simulink model "robot"  (R2014b)
settings: Solver=ode3  StartTime=0.0  StopTime=inf  RelTol=1e-3
libraries: vexarmcortexlib x28
settings Model: Creator=Chase  LastModifiedBy=Chase
settings OptimizationCC: OptimizeModelRefInitCode=on  LifeSpan=Inf  MaxStackSize=64
settings HardwareCC: ProdLargestAtomicInteger=Long  ProdLargestAtomicFloat=Double  ProdEndianess=LittleEndian  ProdHWDeviceType=ARM Compatible->ARM Cortex
settings RTWCC: SystemTargetFile=ert.tlc  TLCOptions=-aInlineSetEventsForThisBaseRateFcn=TLC_FALSE -aSuppressMultiTaskScheduler=TLC_FALSE  TemplateMakefile=ert_default_tmf  Description=Embedded Coder  ProcessScript=ert_make_rtw_hook  Toolchain=GNU Tools for VEX ARM Cortex
settings CodeAppCC: IgnoreCustomStorageClasses=off
settings ERTTargetCC: CodeReplacementLibrary=GCC ARM Cortex-M3

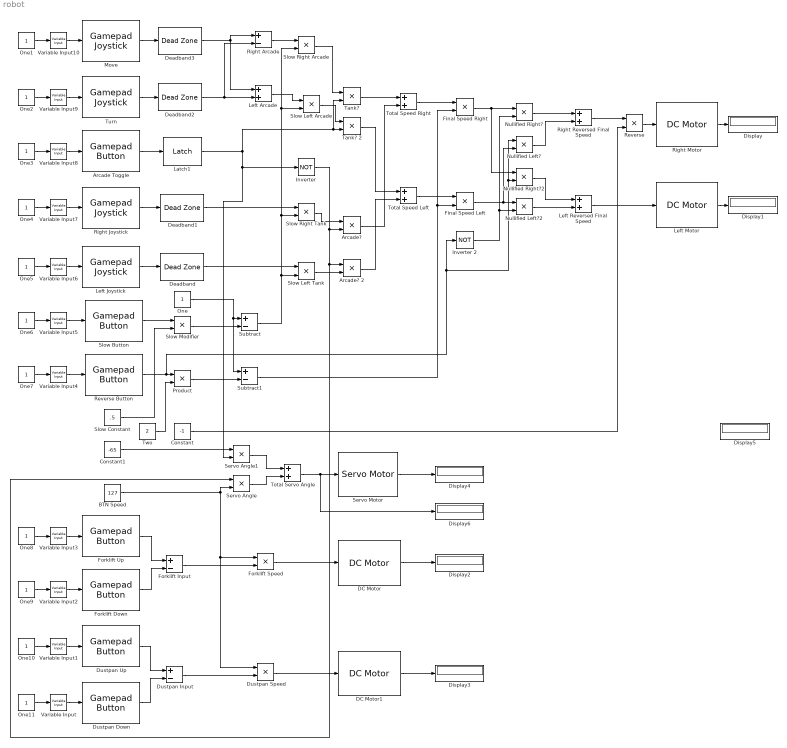
== system robot ==
  Arcade Toggle : vexarmcortexlib/Gamepad Button  joystick=1  chan=5  button56=Down  button78=Right
  Arcade? : Product  RndMeth=Zero
  Arcade? 2 : Product  RndMeth=Zero
  "BTN Speed " : Constant  Value=127
  Constant : Constant  Value=-1
  Constant1 : Constant  Value=-65
  DC Motor : vexarmcortexlib/DC Motor  motor=3  scaleFactor=1/13.5
  DC Motor1 : vexarmcortexlib/DC Motor  motor=8  scaleFactor=1/13.5
  Deadband{,1..3} (4 alike) : DeadZone  LowerValue=-10  UpperValue=10  SaturateOnIntegerOverflow=on
  Display{,1..6} (7 alike) : Display
  Dustpan Down : vexarmcortexlib/Gamepad Button  joystick=1  chan=7  button56=Down  button78=Down
  Dustpan Input : Sum  Inputs=+-
  Dustpan Speed : Product  RndMeth=Zero
  Dustpan Up : vexarmcortexlib/Gamepad Button  joystick=1  chan=7  button56=Down  button78=Up
  Final Speed Left : Product  RndMeth=Zero
  Final Speed Right : Product  RndMeth=Zero
  Forklift Down : vexarmcortexlib/Gamepad Button  joystick=1  chan=8  button56=Up  button78=Down
  Forklift Input : Sum  Inputs=+-
  Forklift Speed : Product  RndMeth=Zero
  Forklift Up : vexarmcortexlib/Gamepad Button  joystick=1  chan=8  button56=Up  button78=Up
  Inverter : Logic  Operator=NOT  AllPortsSameDT=off  OutDataTypeStr=boolean
  "Inverter 2 " : Logic  Operator=NOT  AllPortsSameDT=off  OutDataTypeStr=boolean
  Latch1 : vexarmcortexlib/Utilities/Latch  output0=off
  Left Arcade : Sum
  Left Joystick : vexarmcortexlib/Gamepad Joystick  joystick=1  chan=3
  Left Motor : vexarmcortexlib/DC Motor  motor=9  scaleFactor=1/13.5
  Left Reversed Final Speed : Sum
  Move : vexarmcortexlib/Gamepad Joystick  joystick=1  chan=3
  Nullified Left? : Product  RndMeth=Zero
  Nullified Left?2 : Product  RndMeth=Zero
  Nullified Right? : Product  RndMeth=Zero
  Nullified Right?2 : Product  RndMeth=Zero
  One{,1..11} (12 alike) : Constant
  Product : Product
  Reverse : Product  RndMeth=Zero
  Reverse Button : vexarmcortexlib/Gamepad Button  joystick=1  chan=6  button56=Up  button78=Right
  Right Arcade : Sum  Inputs=+-
  Right Joystick : vexarmcortexlib/Gamepad Joystick  joystick=1  chan=2
  Right Motor : vexarmcortexlib/DC Motor  motor=2  scaleFactor=1/13.5
  Right Reversed Final Speed : Sum
  Servo Angle : Product  RndMeth=Zero
  Servo Angle1 : Product  RndMeth=Zero
  Servo Motor : vexarmcortexlib/Servo Motor  motor=7  scaleFactor=90/127
  Slow Button : vexarmcortexlib/Gamepad Button  joystick=1  chan=5  button56=Up  button78=Up
  Slow Constant : Constant  Value=.5
  Slow Left Arcade : Product  RndMeth=Zero
  Slow Left Tank : Product  RndMeth=Zero
  Slow Modifier : Product  RndMeth=Zero
  Slow Right Arcade : Product  RndMeth=Zero
  Slow Right Tank : Product  RndMeth=Zero
  Subtract : Sum  Inputs=+-
  Subtract1 : Sum  Inputs=+-
  Tank? : Product  RndMeth=Zero
  Tank? 2 : Product  RndMeth=Zero
  Total Servo Angle : Sum
  Total Speed Left : Sum
  Total Speed Right : Sum
  Turn : vexarmcortexlib/Gamepad Joystick  joystick=1  chan=1
  Two : Constant  Value=2
  Variable Input{,1..5,8} (7 alike) : vexarmcortexlib/Utilities/Variable Input  low=0  gain=0  high=1
  Variable Input{6..7,9..10} (4 alike) : vexarmcortexlib/Utilities/Variable Input  low=-127  gain=0  high=127
  wires:
  Right Motor/1 -> Display/1
  Left Motor/1 -> Display1/1
  Left Joystick/1 -> Deadband/1
  Right Joystick/1 -> Deadband1/1
  Variable Input2/1 -> Forklift Down/1
  Variable Input3/1 -> Forklift Up/1
  Forklift Up/1 -> Forklift Input/1
  Forklift Down/1 -> Forklift Input/2
  Variable Input1/1 -> Dustpan Up/1
  Variable Input/1 -> Dustpan Down/1
  Dustpan Up/1 -> Dustpan Input/1
  Dustpan Down/1 -> Dustpan Input/2
  Latch1/1 -> Servo Angle1/2, Inverter/1, Tank?/2, Tank? 2/2
  Arcade Toggle/1 -> Latch1/1
  Variable Input8/1 -> Arcade Toggle/1
  Move/1 -> Deadband3/1
  Turn/1 -> Deadband2/1
  Deadband3/1 -> Right Arcade/1, Left Arcade/1
  Deadband2/1 -> Left Arcade/2, Right Arcade/2
  "BTN Speed "/1 -> Servo Angle/2, Dustpan Speed/1, Forklift Speed/1
  Forklift Input/1 -> Forklift Speed/2
  Dustpan Input/1 -> Dustpan Speed/2
  Dustpan Speed/1 -> DC Motor1/1
  Forklift Speed/1 -> DC Motor/1
  DC Motor/1 -> Display2/1
  DC Motor1/1 -> Display3/1
  Variable Input5/1 -> Slow Button/1
  Slow Button/1 -> Slow Modifier/1
  Slow Constant/1 -> Slow Modifier/2
  Left Arcade/1 -> Slow Left Arcade/1
  Right Arcade/1 -> Slow Right Arcade/1
  Deadband1/1 -> Slow Right Tank/1
  Deadband/1 -> Slow Left Tank/1
  Variable Input10/1 -> Move/1
  Variable Input9/1 -> Turn/1
  Variable Input7/1 -> Right Joystick/1
  Variable Input6/1 -> Left Joystick/1
  Slow Left Tank/1 -> Arcade? 2/2
  Slow Left Arcade/1 -> Tank? 2/1
  Slow Right Arcade/1 -> Tank?/1
  Inverter/1 -> Arcade?/2, Servo Angle/1, Arcade? 2/1
  Slow Right Tank/1 -> Arcade?/1
  Arcade?/1 -> Total Speed Right/2
  Arcade? 2/1 -> Total Speed Left/2
  Tank? 2/1 -> Total Speed Left/1
  Tank?/1 -> Total Speed Right/1
  Variable Input4/1 -> Reverse Button/1
  Total Speed Left/1 -> Final Speed Left/1
  Total Speed Right/1 -> Final Speed Right/1
  Slow Modifier/1 -> Subtract/2
  One/1 -> Subtract1/1, Subtract/1
  Subtract/1 -> Slow Right Tank/2, Slow Right Arcade/2, Slow Left Arcade/2, Slow Left Tank/2
  Reverse Button/1 -> "Inverter 2 "/1, Nullified Right?2/2, Nullified Left?/1, Product/1
  Two/1 -> Product/2
  Product/1 -> Subtract1/2
  Subtract1/1 -> Final Speed Right/2, Final Speed Left/2
  "Inverter 2 "/1 -> Nullified Right?/2, Nullified Left?2/2
  Final Speed Left/1 -> Nullified Left?2/1, Nullified Left?/2
  Final Speed Right/1 -> Nullified Right?2/1, Nullified Right?/1
  Nullified Right?/1 -> Right Reversed Final Speed/1
  Nullified Left?/1 -> Right Reversed Final Speed/2
  Nullified Right?2/1 -> Left Reversed Final Speed/1
  Nullified Left?2/1 -> Left Reversed Final Speed/2
  Constant/1 -> Reverse/2
  One1/1 -> Variable Input10/1
  One2/1 -> Variable Input9/1
  One3/1 -> Variable Input8/1
  One4/1 -> Variable Input7/1
  One5/1 -> Variable Input6/1
  One6/1 -> Variable Input5/1
  One7/1 -> Variable Input4/1
  One8/1 -> Variable Input3/1
  One9/1 -> Variable Input2/1
  One10/1 -> Variable Input1/1
  One11/1 -> Variable Input/1
  Reverse/1 -> Right Motor/1
  Right Reversed Final Speed/1 -> Reverse/1
  Left Reversed Final Speed/1 -> Left Motor/1
  Servo Motor/1 -> Display4/1
  Constant1/1 -> Servo Angle1/1
  Servo Angle1/1 -> Total Servo Angle/1
  Servo Angle/1 -> Total Servo Angle/2
  Total Servo Angle/1 -> Display6/1, Servo Motor/1
